simulink model "Clark_transformation"  (R2019a)
settings: Solver=VariableStepAuto  StartTime=0.0  StopTime=1  MaxStep=1e-4  RelTol=1e-3
libraries: powerlib_meascontrol x1
settings Model: Creator=Deepak  LastModifiedBy=Deepak

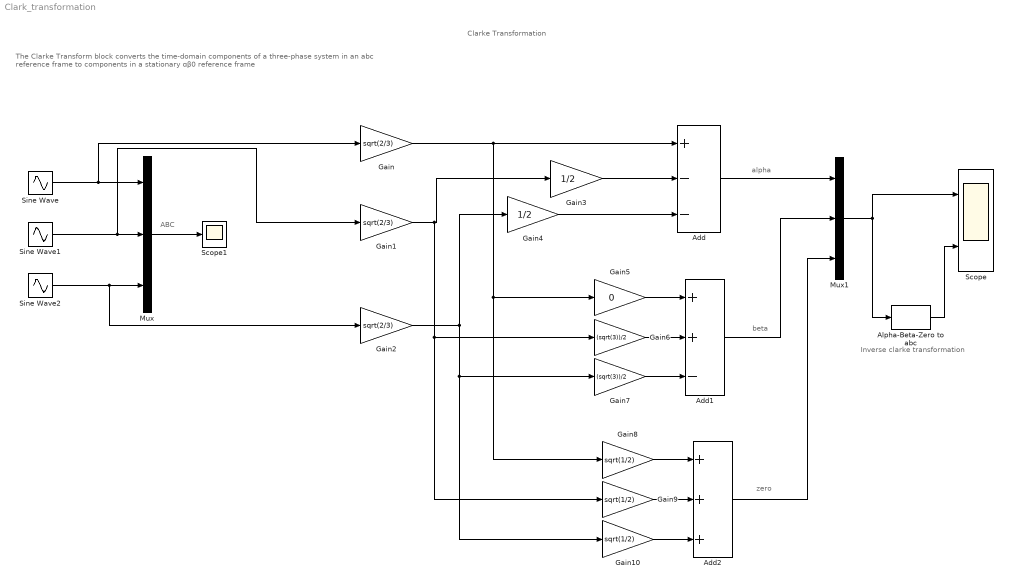
== system Clark_transformation ==
  note: Inverse clarke transformation
  note: ABC
  note: zero
  note: beta
  note: alpha
  note: Clarke Transformation
  note: The Clarke Transform block converts the time-domain components of a three-phase system in an abc reference frame to components in a stationary ɑβ0 reference frame
  Add : Sum  Inputs=+--
  Add1 : Sum  Inputs=++-
  Add2 : Sum  Inputs=+++
  Alpha-Beta-Zero to abc : powerlib_meascontrol/Transformations/Alpha-Beta-Zero to abc
      settings: SourceProductName=Simscape Electrical  SourceProductBaseCode=PS
  Gain : Gain  Gain=sqrt(2/3)
  Gain1 : Gain  Gain=sqrt(2/3)
  Gain10 : Gain  Gain=sqrt(1/2)
  Gain2 : Gain  Gain=sqrt(2/3)
  Gain3 : Gain  Gain=1/2
  Gain4 : Gain  Gain=1/2
  Gain5 : Gain  Gain=0
  Gain6 : Gain  Gain=(sqrt(3))/2
  Gain7 : Gain  Gain=(sqrt(3))/2
  Gain8 : Gain  Gain=sqrt(1/2)
  Gain9 : Gain  Gain=sqrt(1/2)
  Mux : Mux  Inputs=3
  Mux1 : Mux  Inputs=3
  Scope : Scope  NumInputPorts=2
  Scope1 : Scope
  Sine Wave : Sin  Amplitude=10  Frequency=50  SampleTime=0
  Sine Wave1 : Sin  Amplitude=10  Frequency=50  Phase=-120*(pi/180)  SampleTime=0
  Sine Wave2 : Sin  Amplitude=10  Frequency=50  Phase=120*(pi/180)  SampleTime=0
  wires:
  Sine Wave/1 -> Gain/1, Mux/1
  Sine Wave2/1 -> Gain2/1, Mux/3
  Gain/1 -> Gain8/1, Gain5/1, Add/1
  Gain3/1 -> Add/2
  Gain4/1 -> Add/3
  Sine Wave1/1 -> Gain1/1, Mux/2
  Gain2/1 -> Gain4/1, Gain10/1, Gain7/1
  Gain1/1 -> Gain9/1, Gain6/1, Gain3/1
  Gain5/1 -> Add1/1
  Gain6/1 -> Add1/2
  Gain7/1 -> Add1/3
  Gain10/1 -> Add2/3
  Gain8/1 -> Add2/1
  Gain9/1 -> Add2/2
  Add/1 -> Mux1/1
  Add1/1 -> Mux1/2
  Add2/1 -> Mux1/3
  Mux1/1 -> Alpha-Beta-Zero to abc/1, Scope/1
  Alpha-Beta-Zero to abc/1 -> Scope/2
  Mux/1 -> Scope1/1
